simulink model "sgMdl_IEC61850_1CLI2SRV"  (R2024b)
settings: Solver=FixedStepAuto  StartTime=0.0  StopTime=inf  RelTol=1e-3  EnableMultiTasking=on
undefined symbols (not defined in the file): GGIO1, LLN0, simpleIOGenericIO
libraries: speedgoatlib_iec61850 x17, slrealtimeutilitieslib x3
Description:
  | IEC 61850 - 1 Client 2 Servers Loopback
settings Model: sg_rtwmakecfg_data=_sg_IO75X_v1_2_0__sg_netxLib_MSVC140_  ModifiedByFormat=Speedgoat  SimulationMode=external  ExtModeEnableFloating=off  Creator=Speedgoat  LastModifiedBy=Speedgoat
settings SolverCC: ConcurrentTasks=on  AlgebraicLoopSolver=TrustRegion  PositivePriorityOrder=on  AutoInsertRateTranBlk=on  InsertRTBMode=Never (minimum delay)
settings DataIOCC: LimitDataPoints=on  SaveFormat=StructureWithTime  ReturnWorkspaceOutputs=off
settings OptimizationCC: BlockReduction=off  BooleanDataType=off  OptimizeBlockIOStorage=off  BufferReuse=off  ReuseModelBlockBuffer=off  GlobalBufferReuse=off  ExpressionFolding=off  LocalBlockOutputs=off  OptimizeDataStoreBuffers=off  BusAssignmentInplaceUpdate=off
settings DebuggingCC: SaveWithParameterizedLinksMsg=none  UnderspecifiedInitializationDetection=Classic  MergeDetectMultiDrivingBlocksExec=none  SignalResolutionControl=TryResolveAllWithWarning  InheritedTsInSrcMsg=none  TasksWithSamePriorityMsg=none  ParameterOverflowMsg=warning  UnconnectedInputMsg=warning  UnconnectedOutputMsg=warning  UnconnectedLineMsg=warning  SFUnexpectedBacktrackingDiag=warning  SFNoUnconditionalDefaultTransitionDiag=warning  SFExecutionAtInitializationDiag=none  ArithmeticOperatorsInVariantConditions=warning
settings HardwareCC: ProdBitPerLong=64  ProdLongLongMode=on  ProdHWDeviceType=Intel->x86-64 (Linux 64)  TargetBitPerPointer=64  TargetBitPerSizeT=64  TargetBitPerPtrDiffT=64  TargetLongLongMode=on  TargetIntDivRoundTo=Zero  TargetEndianess=LittleEndian  TargetWordSize=64  TargetHWDeviceType=MATLAB Host
settings ModelReferenceCC: EnableRefExpFcnMdlSchedulingChecks=on  PropagateSignalLabelsOutOfModel=off
settings SFSimCC: SimUseLocalCustomCode=off  CustomCodeUndefinedFunction=UseInterfaceOnly
settings RTWCC: Description=Speedgoat Real-Time Target Machine  SystemTargetFile=speedgoat.tlc  TemplateMakefile=slrealtime_default_tmf  RetainRTWFile=on  RTWUseLocalCustomCode=off  Toolchain=Simulink Real-Time Toolchain  BuildConfiguration=Faster Runs  TargetLang=C++  GPUComputeCapability=3.5  DLArmComputeVersion=19.05
settings CodeAppCC: StateflowObjectComments=on
settings SimulinkRealTimeTargetCC: SubcomponentCodeInterfacePackaging=Reusable function  InstructionSetFMA=off  LogToMDFFile=off  SLRTFileLogMaxRuns=10
settings ConfigComp: CovMetricSettings=dw  CovSaveCumulativeToWorkspaceVar=on  CovSaveSingleToWorkspaceVar=on  CovExternalEMLEnable=off  CovBoundaryAbsTol=1.0e-5

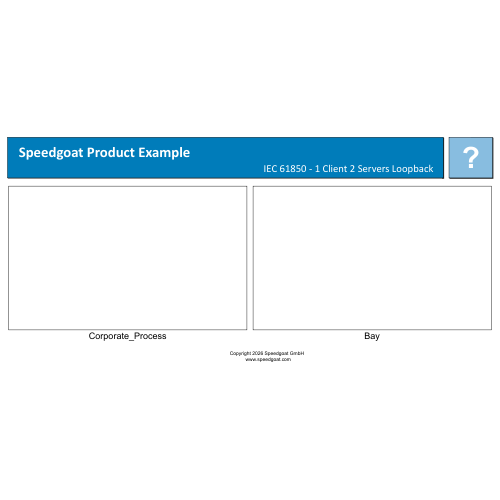
[thumbnail: Simulink's stored preview of the top-level diagram]
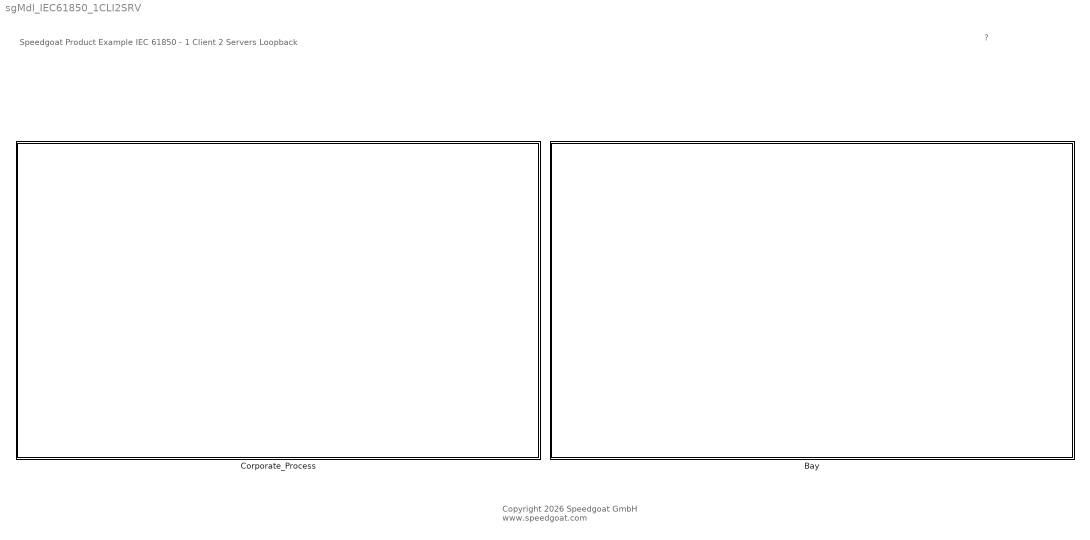
== system sgMdl_IEC61850_1CLI2SRV ==
  note: Speedgoat Product Example
      | IEC 61850 - 1 Client 2 Servers Loopback
  note: ?
  note: Copyright 2026 Speedgoat GmbH
      |  www.speedgoat.com
  Bay : Subsystem
  Corporate_Process : Subsystem

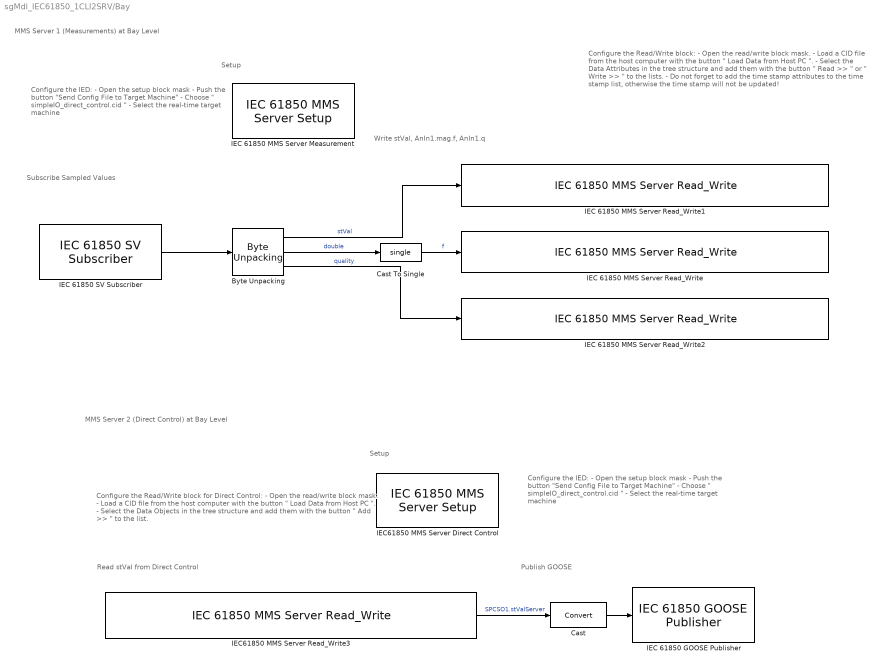
== system sgMdl_IEC61850_1CLI2SRV/Bay ==
  note: Setup
  note: Setup
  note: Write stVal, AnIn1.mag.f, AnIn1.q
  note: Subscribe Sampled Values
  note: Read stVal from Direct Control
  note: Publish GOOSE
  note: MMS Server 2 (Direct Control) at Bay Level
  note: MMS Server 1 (Measurements) at Bay Level
  note: Configure the IED:
      | - Open the setup block mask
      | - Push the button "Send Config File to Target Machine"
      | - Choose " simpleIO_direct_control.cid "
      | - Select the real-time target machine
  note: Configure the IED:
      | - Open the setup block mask
      | - Push the button "Send Config File to Target Machine"
      | - Choose " simpleIO_direct_control.cid "
      | - Select the real-time target machine
  note: Configure the Read/Write block:
      | - Open the read/write block mask.
      | - Load a CID file from the host computer with the button
      | " Load Data from Host PC ".
      | - Select the Data Attributes in the tree structure and add them with the button
      | " Read >> " or " Write >> " to the lists.
      | - Do not forget to add the time stamp attributes to the time stamp list,
      | otherwise the time stamp will not be updated!
  note: Configure the Read/Write block for Direct Control:
      | - Open the read/write block mask.
      | - Load a CID file from the host computer with the button
      | " Load Data from Host PC ".
      | - Select the Data Objects in the tree structure and add them with the button
      | " Add >> " to the list.
  Byte Unpacking : slrealtimeutilitieslib/Byte Unpacking  MaskUnpackedDataTypes={'uint8', 'double', 'uint32'}  MaskUnpackedDataSizes={[1],[1],[1]}  MaskAlignment=1
  Cast : DataTypeConversion  SaturateOnIntegerOverflow=off  RndMeth=Floor
  Cast To Single : DataTypeConversion  OutDataTypeStr=single  SaturateOnIntegerOverflow=off  RndMeth=Floor
  IEC 61850 GOOSE Publisher : speedgoatlib_iec61850/GOOSE/IEC 61850 GOOSE Publisher  ServerID=0  EthernetPort_Param='ETH1'  DataType_Param=Int8  BaseIntervall_Param=100  SampleTime=-1  MACAddress_Param='00:01:29:ac:1a:c6'  AppID=4096  VLANID=0  VLAN_Prio=4  GoCbRef_Param='simpleIOGenericIO/LLN0$GO$gcbEvents'  DataSetRef_Param='simpleIOGenericIO/LLN0$GO$Events'  GoID_Param='simpleIOGenericIO/LLN0$GO$gcbEvents'
      settings: SourceProductName=IEC 61850
      settings: AttributesFormatString=|
      | Destination MAC Address:
      | %<MACAddress_Param>
  IEC 61850 MMS Server Measurement : speedgoatlib_iec61850/Server/IEC 61850 MMS Server Setup  ServerID=1  IpAddrStr=IP_Server_01  TcpPort=102  Authenticate=off  Enabler='speedgoat'  KeepAlive=0  SampleTime=-1  ST=off  MX=on  SP=off  SV=off  CF=off  DC=on  SG=off  SE=off  SR=off  OR=off  BL=off  EX=off  CO=off  US=off  MS=off  RP=off  BR=off  LG=off  GO=off
      settings: AttributesFormatString=%<IpAddrStr>  SourceProductName=IEC 61850
  IEC 61850 MMS Server Read_Write : speedgoatlib_iec61850/Server/IEC 61850 MMS Server Read_Write  StationID=1  SampleTime=-1  ReadDimension=0  WriteDimension=1  TimeDimension=1  ControlDimension=0  ReadAttributes={''}  WriteAttributes={''}  TimeAttributes={''}  WriteArea=simpleIOGenericIO/GGIO1.MX.AnIn1.mag.f  TimeArea=simpleIOGenericIO/GGIO1.MX.AnIn1.t  DataType=single
      settings: AttributesFormatString=Port Data Type: %<DataType>  SourceProductName=IEC 61850
  IEC 61850 MMS Server Read_Write1 : speedgoatlib_iec61850/Server/IEC 61850 MMS Server Read_Write  StationID=1  SampleTime=-1  ReadDimension=0  WriteDimension=1  TimeDimension=1  ControlDimension=0  ReadAttributes={''}  WriteAttributes={''}  TimeAttributes={''}  WriteArea=simpleIOGenericIO/GGIO1.ST.Ind1.stVal  TimeArea=simpleIOGenericIO/GGIO1.ST.Ind1.t  DataType=uint8
      settings: AttributesFormatString=Port Data Type: %<DataType>  SourceProductName=IEC 61850
  IEC 61850 MMS Server Read_Write2 : speedgoatlib_iec61850/Server/IEC 61850 MMS Server Read_Write  StationID=1  SampleTime=-1  ReadDimension=0  WriteDimension=1  TimeDimension=0  ControlDimension=0  ReadAttributes={''}  WriteAttributes={''}  TimeAttributes={''}  WriteArea=simpleIOGenericIO/GGIO1.MX.AnIn1.q  DataType=uint32
      settings: AttributesFormatString=Port Data Type: %<DataType>  SourceProductName=IEC 61850
  IEC 61850 SV Subscriber : speedgoatlib_iec61850/Sampled Values/IEC 61850 SV Subscriber  ServerID=0  EthernetPort_Param='ETH1'  DataType_Param=Int8  DataBytes_Param=13  SampleTime=-1  MACAddress_Param='00:01:29:88:60:76'  AppID=16384
      settings: SourceProductName=IEC 61850
      settings: AttributesFormatString=|
      | Destination MAC Address:
      | %<MACAddress_Param>
  IEC61850 MMS Server Direct Control : speedgoatlib_iec61850/Server/IEC 61850 MMS Server Setup  ServerID=2  IpAddrStr=IP_Server_02  TcpPort=102  Authenticate=off  Enabler='speedgoat'  KeepAlive=0  SampleTime=-1  ST=off  MX=on  SP=off  SV=off  CF=off  DC=off  SG=off  SE=off  SR=off  OR=off  BL=off  EX=off  CO=off  US=off  MS=off  RP=off  BR=off  LG=off  GO=off
      settings: AttributesFormatString=%<IpAddrStr>  SourceProductName=IEC 61850
  IEC61850 MMS Server Read_Write3 : speedgoatlib_iec61850/Server/IEC 61850 MMS Server Read_Write  StationID=2  SampleTime=-1  ReadDimension=1  WriteDimension=0  TimeDimension=2  ControlDimension=1  ReadAttributes={''}  WriteAttributes={''}  TimeAttributes={''}  ReadArea=simpleIOGenericIO/GGIO1.ST.SPCSO1.stVal  TimeArea=simpleIOGenericIO/GGIO1.MX.AnIn3.t simpleIOGenericIO/GGIO1.MX.AnIn4.t  ControlArea=simpleIOGenericIO/GGIO1.CO.SPCSO1  DataType=boolean
      settings: AttributesFormatString=Port Data Type: %<DataType>  SourceProductName=IEC 61850
  wires:
  Byte Unpacking/1 -> IEC 61850 MMS Server Read_Write1/1  "stVal"
  Byte Unpacking/3 -> IEC 61850 MMS Server Read_Write2/1  "quality"
  Byte Unpacking/2 -> Cast To Single/1  "double"
  IEC 61850 SV Subscriber/1 -> Byte Unpacking/1
  Cast To Single/1 -> IEC 61850 MMS Server Read_Write/1  "f"
  IEC61850 MMS Server Read_Write3/1 -> Cast/1  "SPCSO1.stValServer"
  Cast/1 -> IEC 61850 GOOSE Publisher/1

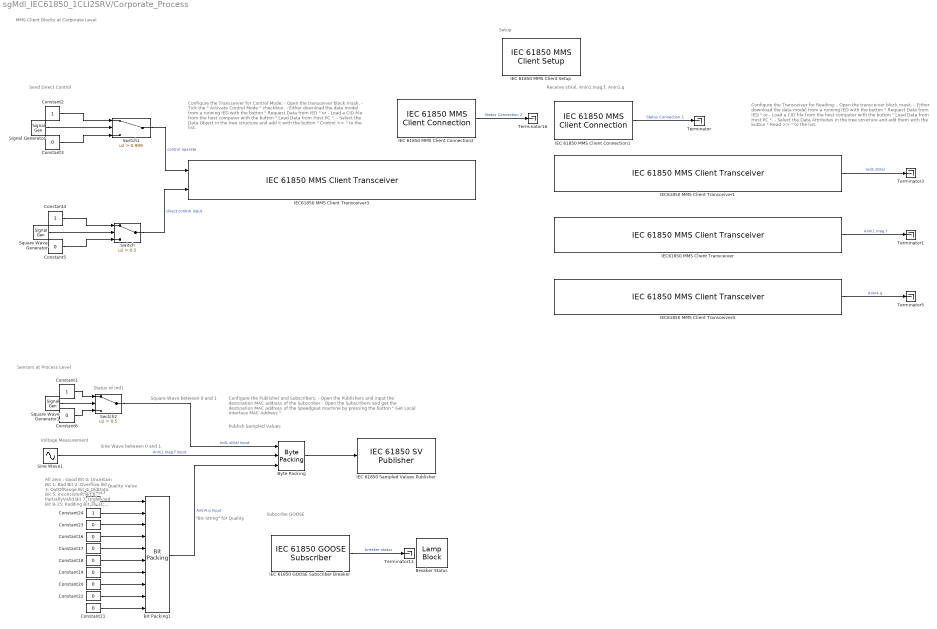
== system sgMdl_IEC61850_1CLI2SRV/Corporate_Process ==
  note: MMS Client Blocks at Corporate Level
  note: Square Wave between 0 and 1
  note: Sine Wave between 0 and 1
  note: Status of Ind1
  note: Voltage Measurement
  note: "Bit-String" for Quality
  note: Quality Value
  note: Sensors at Process Level
  note: All zero : Good
      |
      | Bit 0: Uncertain
      |
      | Bit 1: Bad
      |
      | Bit 2: Overflow
      |
      | Bit 3: OutOfRange
      |
      | Bit 4: OldData
      |
      | Bit 5: Inconsistent
      |
      | Bit 6: PartiallyValid
      |
      | Bit 7: Undefined
      |
      | Bit 8-15: Padding
      |
      | Bit 16-31: Padding
  note: Setup
  note: Send Direct Control
  note: Receive stVal, AnIn1.mag.f, AnIn1.q
  note: Publish Sampled Values
  note: Subscribe GOOSE
  note: Configure the Transceiver for Control Mode:
      | - Open the transceiver block mask.
      | - Tick the " Activate Control Mode " checkbox.
      | - Either download the data model from a running IED with the button
      | " Request Data from IED " or
      | - Load a CID file from the host computer with the button
      | " Load Data from Host PC ".
      | - Select the Data Object in the tree structure and add it with the button
      | " Control >> " to the list.
  note: Configure the Transceiver for Reading:
      | - Open the transceiver block mask.
      | - Either download the data model from a running IED with the button
      | " Request Data from IED " or
      | - Load a CID file from the host computer with the button
      | " Load Data from Host PC ".
      | - Select the Data Attributes in the tree structure and add them with the button
      | " Read >> " to the list.
  note: Configure the Publisher and Subscribers:
      | - Open the Publishers and input the destination MAC address of the Subscriber
      | - Open the Subscribers and get the destination MAC address of the Speedgoat machine by pressing the button " Get Local Interface MAC Address "
  Bit Packing1 : slrealtimeutilitieslib/Bit Packing  MaskBitPatterns={[0],[1],[2],[3],[4],[5],[6],[7],[8:15],[16:31]}  MaskPackDataType=uint32  MaskPackDataSize=[1]
  Breaker Status : LampBlock  LabelPosition=Hide
  Byte Packing : slrealtimeutilitieslib/Byte Packing  MaskPackedDataType=int8  MaskUnpackedDataTypes={'uint8', 'double', 'uint32'}  MaskAlignment=1
  Constant1 : Constant  OutDataTypeStr=uint8
  Constant{16..20,23,25} (7 alike) : Constant  Value=0  OutDataTypeStr=boolean  SampleTime=-1
  Constant2 : Constant  OutDataTypeStr=boolean
  Constant21 : Constant  Value=0  OutDataTypeStr=uint16  SampleTime=-1
  Constant22 : Constant  Value=0  OutDataTypeStr=uint8  SampleTime=-1
  Constant24 : Constant  OutDataTypeStr=boolean  SampleTime=-1
  Constant3 : Constant  Value=0  OutDataTypeStr=boolean
  Constant4 : Constant  OutDataTypeStr=boolean
  Constant5 : Constant  Value=0  OutDataTypeStr=boolean
  Constant6 : Constant  Value=0  OutDataTypeStr=uint8
  IEC 61850 GOOSE Subscriber Breaker : speedgoatlib_iec61850/GOOSE/IEC 61850 GOOSE Subscriber  ServerID=0  EthernetPort_Param='ETH1'  DataType_Param=Int8  DataBytes_Param=1  SampleTime=-1  MACAddress_Param='00:01:29:ac:1a:c6'  AppID=4096  GoCbRef_Param='simpleIOGenericIO/LLN0$GO$gcbEvents'
      settings: SourceProductName=IEC 61850
      settings: AttributesFormatString=|
      | Destination MAC Address:
      | %<MACAddress_Param>
  IEC 61850 MMS Client Connection1 : speedgoatlib_iec61850/Client/IEC 61850 MMS Client Connection  IsConnection=1  ClientID=20  ConnectionID=1  remoteipAddrStr=IP_Server_01  remoteTCPPort=102  SampleTime=-1  enaReport=off  ReportArea=simpleIOGenericIO/LLN0.RP.EventsRCB01  Authenticate=off  Enabler='speedgoat'  AP_Title='1,3,9999,33'  AE_Qualifier=33
      settings: SourceProductName=IEC 61850
      settings: AttributesFormatString=|
      | Remote IP: %<remoteipAddrStr>
      | Remote TCP Port: %<remoteTCPPort>
  IEC 61850 MMS Client Connection2 : speedgoatlib_iec61850/Client/IEC 61850 MMS Client Connection  IsConnection=1  ClientID=20  ConnectionID=2  remoteipAddrStr=IP_Server_02  remoteTCPPort=102  SampleTime=-1  enaReport=off  ReportArea=simpleIOGenericIO/LLN0.RP.EventsRCB01  Authenticate=off  Enabler='speedgoat'  AP_Title='1,3,9999,33'  AE_Qualifier=33
      settings: SourceProductName=IEC 61850
      settings: AttributesFormatString=|
      | Remote IP: %<remoteipAddrStr>
      | Remote TCP Port: %<remoteTCPPort>
  IEC 61850 MMS Client Setup : speedgoatlib_iec61850/Client/IEC 61850 MMS Client Setup  IsSetup=1  ClientID=20  locIpAddrStr=IP_Client_00  SampleTime=-1
      settings: SourceProductName=IEC 61850
  IEC 61850 Sampled Values Publisher : speedgoatlib_iec61850/Sampled Values/IEC 61850 SV Publisher  ServerID=2  EthernetPort_Param='ETH1'  DataType_Param=Int8  EnaTimeStamp=on  PollingTime=10000  SampleTime=-1  TimeStampCB=on  ASDU_Param='VoltageMUX1'  MACAddress_Param='00:01:29:88:60:76'  AppID=16384  VLANID=0  VLAN_Prio=4
      settings: SourceProductName=IEC 61850
      settings: AttributesFormatString=|
      | Destination MAC Address:
      | %<MACAddress_Param>
  IEC61850 MMS Client Transceiver : speedgoatlib_iec61850/Client/IEC 61850 MMS Client Transceiver  StationID=20  ConnectionID=1  PollIntervall=50  SampleTime=-1  ReadDimension=1  WriteDimension=0  ControlDimension=0  ReadAttributes={''}  WriteAttributes={''}  ReadArea=simpleIOGenericIO/GGIO1.MX.AnIn1.mag.f  CtrlMode_Param=off  CtrlTest_Param=off  DataType=single  ConfigPath=0  ConfigHistory=0
      settings: SourceProductName=IEC 61850
      settings: AttributesFormatString=|
      | Port Data Type:
      | %<DataType>
  IEC61850 MMS Client Transceiver1 : speedgoatlib_iec61850/Client/IEC 61850 MMS Client Transceiver  StationID=20  ConnectionID=1  PollIntervall=10  SampleTime=-1  ReadDimension=1  WriteDimension=0  ControlDimension=0  ReadAttributes={''}  WriteAttributes={''}  ReadArea=simpleIOGenericIO/GGIO1.ST.Ind1.stVal  CtrlMode_Param=off  CtrlTest_Param=off  DataType=int8  ConfigPath=C:\svn\speedgoatlib\product_examples\IEC61850\IEC61850_files\simpleIO_direct_control.cid  ConfigHistory=0
      settings: SourceProductName=IEC 61850
      settings: AttributesFormatString=|
      | Port Data Type:
      | %<DataType>
  IEC61850 MMS Client Transceiver3 : speedgoatlib_iec61850/Client/IEC 61850 MMS Client Transceiver  StationID=20  ConnectionID=2  PollIntervall=1  SampleTime=-1  ReadDimension=0  WriteDimension=0  ControlDimension=1  ReadAttributes={''}  WriteAttributes={''}  ControlArea=simpleIOGenericIO/GGIO1.SPCSO1  CtrlMode_Param=on  CtrlTest_Param=off  DataType=boolean  ConfigPath=0  ConfigHistory=0
      settings: SourceProductName=IEC 61850
      settings: AttributesFormatString=|
      | Port Data Type:
      | %<DataType>
  IEC61850 MMS Client Transceiver4 : speedgoatlib_iec61850/Client/IEC 61850 MMS Client Transceiver  StationID=20  ConnectionID=1  PollIntervall=1000  SampleTime=-1  ReadDimension=1  WriteDimension=0  ControlDimension=0  ReadAttributes={''}  WriteAttributes={''}  ReadArea=simpleIOGenericIO/GGIO1.MX.AnIn1.q  CtrlMode_Param=off  CtrlTest_Param=off  DataType=bit string (uint32)  ConfigPath=0  ConfigHistory=0
      settings: SourceProductName=IEC 61850
      settings: AttributesFormatString=|
      | Port Data Type:
      | %<DataType>
  Signal Generator : SignalGenerator  Frequency=1/14.5
  Sine Wave1 : Sin  Phase=50
  Square Wave Generator : SignalGenerator  WaveForm=square  Frequency=1/2
  Square Wave Generator1 : SignalGenerator  WaveForm=square  Frequency=1/2
  Switch : Switch  Criteria=u2 > Threshold  Threshold=0.5  SaturateOnIntegerOverflow=off  InputSameDT=off
  Switch1 : Switch  Criteria=u2 > Threshold  Threshold=0.999  SaturateOnIntegerOverflow=off  InputSameDT=off
  Switch2 : Switch  Criteria=u2 > Threshold  Threshold=0.5  OutDataTypeStr=Inherit: Inherit via back propagation  SaturateOnIntegerOverflow=off  InputSameDT=off
  Terminator{,1,3,5,11,16} (6 alike) : Terminator
  wires:
  IEC 61850 MMS Client Connection1/1 -> Terminator/1  "Status Connection 1"
  IEC61850 MMS Client Transceiver/1 -> Terminator1/1  "AnIn1.mag.f"
  IEC61850 MMS Client Transceiver4/1 -> Terminator5/1  "AnIn4.q"
  Switch/1 -> IEC61850 MMS Client Transceiver3/2  "direct control input"
  Constant5/1 -> Switch/3
  Constant4/1 -> Switch/1
  IEC 61850 MMS Client Connection2/1 -> Terminator16/1  "Status Connection 2"
  Switch1/1 -> IEC61850 MMS Client Transceiver3/1  "control operate"
  IEC61850 MMS Client Transceiver1/1 -> Terminator3/1  "Ind1.stVal"
  Square Wave Generator/1 -> Switch/2
  Signal Generator/1 -> Switch1/2
  Constant2/1 -> Switch1/1
  Constant3/1 -> Switch1/3
  Constant20/1 -> Bit Packing1/8
  Constant17/1 -> Bit Packing1/5
  Sine Wave1/1 -> Byte Packing/2  "AnIn1.mag.f Input"
  Constant22/1 -> Bit Packing1/9
  Constant24/1 -> Bit Packing1/2
  Constant21/1 -> Bit Packing1/10
  Constant18/1 -> Bit Packing1/6
  Constant16/1 -> Bit Packing1/4
  Constant25/1 -> Bit Packing1/1
  Switch2/1 -> Byte Packing/1  "Ind1.stVal Input"
  Constant23/1 -> Bit Packing1/3
  IEC 61850 GOOSE Subscriber Breaker/1 -> Terminator11/1  "breaker status"
  Byte Packing/1 -> IEC 61850 Sampled Values Publisher/1
  Constant19/1 -> Bit Packing1/7
  Bit Packing1/1 -> Byte Packing/3  "AnIn4.q Input"
  Constant6/1 -> Switch2/3
  Constant1/1 -> Switch2/1
  Square Wave Generator1/1 -> Switch2/2
